simulink model "DC_lead_compensator_R2018a"  (R2018a)
settings: Solver=VariableStepAuto  StartTime=0.0  StopTime=0.5  MaxStep=1e-4  RelTol=1e-3
values from neighbouring files (symbols this model uses):
  alphad = 4    [DC_parameters_facit.m]
  b = 20    [DC_SIMC.m]    (also in DC_SIMC_facit.m; DC_parameters.m; DC_parameters_facit.m)
  gr = 200    [DC_SIMC.m]    (also in DC_SIMC_facit.m; DC_parameters.m; DC_parameters_facit.m)
  J = 50*1.5^2    (= 112.5)    [DC_SIMC.m]    (also in DC_SIMC_facit.m; DC_parameters.m; DC_parameters_facit.m)
  K = 2.24/k1/taudc    (= 27893.798051)    [DC_parameters_facit.m]    (also in antenna_lead_lag_51.m = 1/abs(evalfr(G, i*w_c))/sqrt(alpha_d))
  k = Vmax / gr / (speed_max*pi/180)    (= 0.954929658551)    [DC_SIMC.m]    (also in DC_SIMC_facit.m; DC_lead_scaling.m = 200; DC_parameters.m; DC_parameters_facit.m)
  k1 = 1/( gr*k + b*R/(gr*k))    (= 0.00522167224505)    [DC_SIMC.m]    (also in DC_SIMC_facit.m; DC_parameters.m; DC_parameters_facit.m)
  L = 4e-3    (= 0.004)    [DC_SIMC.m]    (also in DC_SIMC_facit.m; DC_parameters.m; DC_parameters_facit.m)
  R = 5    [DC_SIMC.m]    (also in DC_SIMC_facit.m; DC_parameters.m; DC_parameters_facit.m)
  taudc = J/((gr*k)^2/R + b)    (= 0.0153790942167)    [DC_SIMC.m]    (also in DC_SIMC_facit.m; DC_parameters.m; DC_parameters_facit.m)
  Td = 0.25*taudc    (= 0.00384477355418)    [DC_parameters_facit.m]    (also in antenna_lead_lag_51.m = 1/(w_c*sqrt(alpha_d)))
settings Model: Creator=kjartan  LastModifiedBy=kjartan
settings DataIOCC: ReturnWorkspaceOutputs=on
settings DebuggingCC: SFMachineParentedDataDiag=error
settings SFSimCC: SimUseLocalCustomCode=on
settings RTWCC: RTWUseLocalCustomCode=on

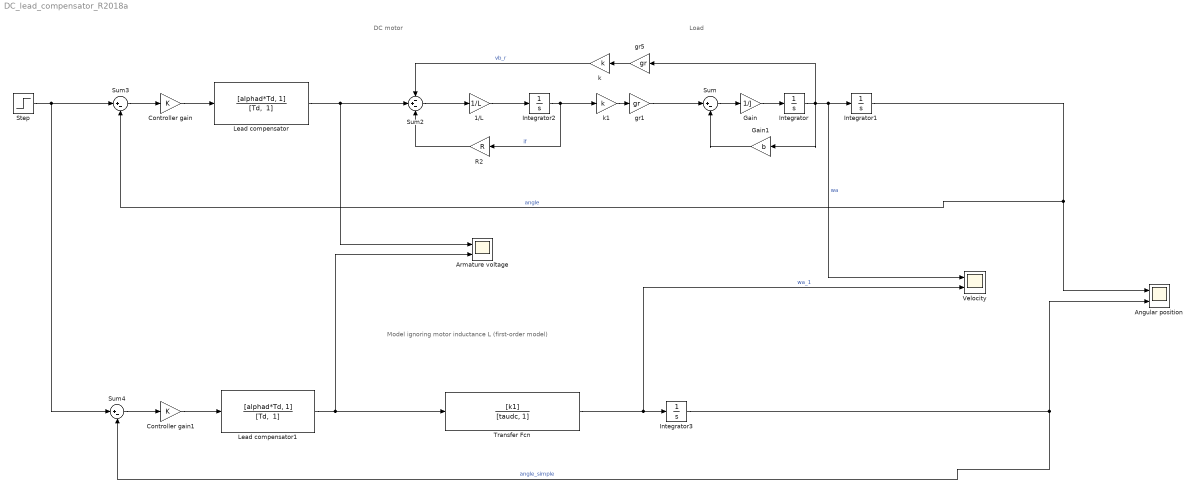
== system DC_lead_compensator_R2018a ==
  note: Model ignoring motor inductance L (first-order model)
  note: Load
  note: DC motor
  1/L : Gain  Gain=1/L
  Angular position : Scope  NumInputPorts=2
  Armature voltage : Scope  NumInputPorts=2
  Controller gain : Gain  Gain=K
  Controller gain1 : Gain  Gain=K
  Gain : Gain  Gain=1/J
  Gain1 : Gain  Gain=b
  Integrator{,1..3} (4 alike) : Integrator
  Lead compensator : TransferFcn  Numerator=[alphad*Td, 1]  Denominator="[Td,  1]"
  Lead compensator1 : TransferFcn  Numerator=[alphad*Td, 1]  Denominator="[Td,  1]"
  R2 : Gain  Gain=R
  Step : Step  Time=0  After=pi/6  SampleTime=0
  Sum : Sum  Inputs=|+-
  Sum2 : Sum  Inputs=-+-
  Sum3 : Sum  Inputs=|+-
  Sum4 : Sum  Inputs=|+-
  Transfer Fcn : TransferFcn  Numerator=[k1]  Denominator=[taudc, 1]
  Velocity : Scope  NumInputPorts=2
  gr1 : Gain  Gain=gr
  gr5 : Gain  Gain=gr
  k : Gain  Gain=k
  k1 : Gain  Gain=k
  wires:
  gr5/1 -> k/1
  R2/1 -> Sum2/3
  Integrator2/1 -> R2/1, k1/1  "if"
  Sum2/1 -> 1/L/1
  k1/1 -> gr1/1
  1/L/1 -> Integrator2/1
  k/1 -> Sum2/1  "vb_r"
  gr1/1 -> Sum/1
  Gain/1 -> Integrator/1
  Integrator/1 -> Gain1/1, gr5/1, Velocity/1, Integrator1/1  "wa"
  Integrator1/1 -> Angular position/1, Sum3/2  "angle"
  Transfer Fcn/1 -> Velocity/2, Integrator3/1  "wa_1"
  Integrator3/1 -> Angular position/2, Sum4/2  "angle_simple"
  Controller gain/1 -> Lead compensator/1
  Sum3/1 -> Controller gain/1
  Step/1 -> Sum4/1, Sum3/1
  Controller gain1/1 -> Lead compensator1/1
  Sum4/1 -> Controller gain1/1
  Lead compensator1/1 -> Transfer Fcn/1, Armature voltage/2
  Lead compensator/1 -> Sum2/2, Armature voltage/1
  Sum/1 -> Gain/1
  Gain1/1 -> Sum/2
